simulink model "sim_all"  (R2020a)
settings: Solver=VariableStepAuto  StartTime=0.0  StopTime=2000  RelTol=1e-3
values from neighbouring files (symbols this model uses):
  a1 = rho * D^4 * alpha1    (= 0.000388302366464)    [data_current.m]
  a2 = -rho * D^3 * alpha2 * (1 - omega)    (= 0.0037030698432)    [data_current.m]
  alpha1 = 0.0113    [data_current.m]
  alpha2 = -0.0091    [data_current.m]
  cornerA = [43.781381 ... (first row only)    [missionC.m]
  cornerB = [43.780975 ... (first row only)    [missionC.m]
  cornerC = [43.780189 ... (first row only)    [missionC.m]
  cornerD = [43.780602 ... (first row only)    [missionC.m]
  ctrl_clockwise = false    [controller.m]
  ctrl_int_bound_or = 0.1    [controller.m]
  ctrl_int_bound_pos = 1    [controller.m]
  ctrl_k_or = 1    [controller.m]
  ctrl_k_pos = 1/3    (= 0.333333333333)    [controller.m]
  ctrl_Ki_vel = 100    [controller.m]
  ctrl_Kp_v_pos = 200    [controller.m]
  ctrl_Kp_vel = 200    [controller.m]
  ctrl_TAM = [  1     1           0           0               0       0;               0     0           1           1               0       0;               0     0           0           0               1       1;               0     0  -(ctrl_r+ctrl_dc)  ctrl_r+ctrl_dc    0       0;               0     0           0           0            -ctrl_r    ctrl_r;           -ctrl_r ctrl_r        0           0       ...(+19 chars)    [controller.m]
  ctrl_Ts = 0.1    [controller.m]
  ctrl_va_uncontrolled = 0.15    [controller.m]
  ctrl_vel_uncontrolled = 0.5    [controller.m]
  D = 0.076    [data_current.m]
  dead_zone_limit = 31.5    [data_current.m]
  depth = 5    [missionC.m]
  distanceFromWall = 8    [missionC.m]
  initInspectedSide = 2    [missionC.m]
  initPoint = [ 43.780796 ... (first row only)    [missionC.m]
  mod_A = pi*mod_R*mod_R    [model.m]
  mod_Cd_F = 0.45    [model.m]
  mod_Cd_M = 0.4    [model.m]
  mod_eta_init = [mod_xNorth; mod_yEast; -mod_zDown; 0; 0; 0]    [model.m]
  mod_g = 9.81    [model.m]
  mod_h0 = 0    [model.m]
  mod_Ixx = mod_Io(1,1)    [model.m]
  mod_Iyy = mod_Io(2,2)    [model.m]
  mod_Izz = mod_Io(3,3)    [model.m]
  mod_Kp_dot = 0    [model.m]
  mod_lat0 = 43.780189    [model.m]
  mod_lon0 = 11.282698    [model.m]
  mod_m = 100    [model.m]
  mod_Mq_dot = mod_Kp_dot    (= 0)    [model.m]
  mod_ni_init = [0; 0; 0; 0; 0; 0]    [model.m]
  mod_Nr_dot = mod_Kp_dot    (= 0)    [model.m]
  mod_p1 = [0; mod_R; 0]    [model.m]
  mod_p2 = [0; -mod_R; 0]    [model.m]
  mod_p3 = [0; 0; (mod_R + mod_z_cm)]    [model.m]
  mod_p4 = [0; 0; -(mod_R + mod_z_cm)]    [model.m]
  mod_p5 = [mod_R; 0; 0]    [model.m]
  mod_p6 = [-mod_R; 0; 0]    [model.m]
  mod_R = ((3*mod_Vol)/(4*pi))^(1/3)    [model.m]
  mod_Rm = (4*mod_R)/(3*pi)    [model.m]
  mod_t1 = [1; 0; 0]    [model.m]
  mod_t2 = [1; 0; 0]    [model.m]
  mod_t3 = [0; 1; 0]    [model.m]
  mod_t4 = [0; 1; 0]    [model.m]
  mod_t5 = [0; 0; 1]    [model.m]
  mod_t6 = [0; 0; 1]    [model.m]
  mod_W = mod_m*mod_g    (= 981)    [model.m]
  mod_Xu_dot = (2/3)*mod_rho_AUV*pi*(mod_R^3)    [model.m]
  mod_Yv_dot = mod_Xu_dot    [model.m]
  mod_z_cm = mod_r_cm(3)    [model.m]
  mod_Zw_dot = mod_Xu_dot    [model.m]
  n_max = 340    [data_current.m]
  nav_DT = 0.1    [navigation.m]
  nav_filter = -1    [data_analysis_simulation_total.m]    (also in navigation.m)
  nav_giro = 2    [navigation.m]
  nav_h0 = 0    [navigation.m]
  nav_lat0 = cornerC(1)    [navigation.m]
  nav_lon0 = cornerC(2)    [navigation.m]
  nav_plane_AB = coefficient_plane(nav_A,nav_B)    [navigation.m]
  nav_plane_BC = coefficient_plane(nav_B,nav_C)    [navigation.m]
  nav_plane_CD = coefficient_plane(nav_C,nav_D)    [navigation.m]
  nav_plane_DA = coefficient_plane(nav_D,nav_A)    [navigation.m]
  nav_resampling = 10000    [navigation.m]
  omega = 0.1    [data_current.m]
  relativeDirection = 30    [missionC.m]
  res_enable_n_eff = 1    [navigation.m]
  rho = 1030    [data_current.m]
  sens_distCM = 0.267    [sensors.m]
  sens_Sample_time_AHRS = 0.1    [sensors.m]
  sens_Sample_time_depth = 0.1    [sensors.m]
  sens_Sample_time_dvl = 0.2    [sensors.m]
  sens_Sample_time_GPS = 1    [sensors.m]
  sens_Sample_time_GYRO = 0.1    [sensors.m]
  sens_Sample_time_sonar = 0.5    [sensors.m]
  sens_threshold = 0.485    [sensors.m]
  sens_Variance_AHRS_pitch = (0.0087)^2    (= 7.569e-05)    [sensors.m]
  sens_Variance_AHRS_roll = (0.0087)^2    (= 7.569e-05)    [sensors.m]
  sens_Variance_AHRS_yaw = (0.0017)^2    (= 2.89e-06)    [sensors.m]
  sens_Variance_depth1 = (0.2)^2    (= 0.04)    [sensors.m]
  sens_Variance_depth2 = (0.4)^2    (= 0.16)    [sensors.m]
  sens_Variance_DVL = (speed*0.03)^2    [sensors.m]
  sens_Variance_GPS = 3    [sensors.m]
  sens_Variance_GYRO = 2.5133e-06    [sensors.m]
  sens_Variance_sonar = 0.05    [sensors.m]
  soglia_or = [0.1, 0.1, 0.1]    [mission.m]
  soglia_orp = 0.1    [mission.m]
  soglia_parete = 0.5    [mission.m]
  soglia_parete_frenata = 0.5    [mission.m]
  soglia_pos = [0.00001, 0.00001, 0.5]    [mission.m]
  soglia_SOS_collisione = 2    [mission.m]
  soglia_SOS_or = [0.25, 0.25, 0.25]    [mission.m]
  soglia_SOS_orp = 0.25    [mission.m]
  soglia_SOS_parete = 1    [mission.m]
  soglia_SOS_pos = [0.00005, 0.00005, 1]    [mission.m]
  soglia_SOS_pos_ris = 2    [mission.m]
  soglia_SOS_vel = 0.2    [mission.m]
  SOS = 0    [mission.m]
  speed = 0.4    [missionC.m]
  stato = 100    [mission.m]
  timer = 40*2    (= 80)    [mission.m]
  Ts_supervisor = 0.1    [mission.m]
undefined symbols (not defined in the file or in its folder): DiscIntNeverNeededParam, nav_A, nav_B, nav_C, nav_D
libraries: simulink x8, cstblocks x6, simulink_extras x1
(part 4 of 8)

== system sim_all/Model/Vehicle Model/P3 ==
  note: n is the rotational speed of the thruster
      | V is the speed component of the water along the thruster axis
      |
      | n is saturated according to data
      | a dead zone is considered according to data
      | the thruster is characterised by 1st order dynamics (tau = 0.2s)
  n3 [rad/s] : Inport
  V3 [m/s] : Inport  Port=2
  Dead Zone : DeadZone  LowerValue=-dead_zone_limit  UpperValue=dead_zone_limit  SaturateOnIntegerOverflow=on
  Propeller3 : MATLAB Function  TreatAsAtomicUnit=on
  Saturation : Saturate  UpperLimit=n_max  LowerLimit=-n_max
  Transfer Fcn : TransferFcn  Denominator=[0.2 1]
  T3 : Outport
  wires:
  V3 [m/s]/1 -> Propeller3/2(V3)
  Saturation/1 -> Propeller3/1(n3)
  Transfer Fcn/1 -> Saturation/1
  Dead Zone/1 -> Transfer Fcn/1
  n3 [rad/s]/1 -> Dead Zone/1
  Propeller3/1(T3) -> T3/1

== system sim_all/Model/Vehicle Model/P4 ==
  note: n is the rotational speed of the thruster
      | V is the speed component of the water along the thruster axis
      |
      | n is saturated according to data
      | a dead zone is considered according to data
      | the thruster is characterised by 1st order dynamics (tau = 0.2s)
  n4 [rad/s] : Inport
  V4 [m/s] : Inport  Port=2
  Dead Zone : DeadZone  LowerValue=-dead_zone_limit  UpperValue=dead_zone_limit  SaturateOnIntegerOverflow=on
  Propeller4 : MATLAB Function  TreatAsAtomicUnit=on
  Saturation : Saturate  UpperLimit=n_max  LowerLimit=-n_max
  Transfer Fcn : TransferFcn  Denominator=[0.2 1]
  T4 : Outport
  wires:
  V4 [m/s]/1 -> Propeller4/2(V4)
  Saturation/1 -> Propeller4/1(n4)
  Transfer Fcn/1 -> Saturation/1
  Dead Zone/1 -> Transfer Fcn/1
  n4 [rad/s]/1 -> Dead Zone/1
  Propeller4/1(T4) -> T4/1

== system sim_all/Model/Vehicle Model/P5 ==
  note: n is the rotational speed of the thruster
      | V is the speed component of the water along the thruster axis
      |
      | n is saturated according to data
      | a dead zone is considered according to data
      | the thruster is characterised by 1st order dynamics (tau = 0.2s)
  n5 [rad/s] : Inport
  V5 [m/s] : Inport  Port=2
  Dead Zone : DeadZone  LowerValue=-dead_zone_limit  UpperValue=dead_zone_limit  SaturateOnIntegerOverflow=on
  Propeller5 : MATLAB Function  TreatAsAtomicUnit=on
  Saturation : Saturate  UpperLimit=n_max  LowerLimit=-n_max
  Transfer Fcn : TransferFcn  Denominator=[0.2 1]
  T5 : Outport
  wires:
  V5 [m/s]/1 -> Propeller5/2(V5)
  Saturation/1 -> Propeller5/1(n5)
  Transfer Fcn/1 -> Saturation/1
  Dead Zone/1 -> Transfer Fcn/1
  n5 [rad/s]/1 -> Dead Zone/1
  Propeller5/1(T5) -> T5/1

== system sim_all/Model/Vehicle Model/P6 ==
  note: n is the rotational speed of the thruster
      | V is the speed component of the water along the thruster axis
      |
      | n is saturated according to data
      | a dead zone is considered according to data
      | the thruster is characterised by 1st order dynamics (tau = 0.2s)
  n6 [rad/s] : Inport
  V6 [m/s] : Inport  Port=2
  Dead Zone : DeadZone  LowerValue=-dead_zone_limit  UpperValue=dead_zone_limit  SaturateOnIntegerOverflow=on
  Propeller6 : MATLAB Function  TreatAsAtomicUnit=on
  Saturation : Saturate  UpperLimit=n_max  LowerLimit=-n_max
  Transfer Fcn : TransferFcn  Denominator=[0.2 1]
  T6 : Outport
  wires:
  V6 [m/s]/1 -> Propeller6/2(V6)
  Saturation/1 -> Propeller6/1(n6)
  Transfer Fcn/1 -> Saturation/1
  Dead Zone/1 -> Transfer Fcn/1
  n6 [rad/s]/1 -> Dead Zone/1
  Propeller6/1(T6) -> T6/1

== system sim_all/PF/Particle Filter/AHRS__check ==
  AHRS_new : Inport
  MATLAB Function4 : MATLAB Function  TreatAsAtomicUnit=on
  Memory4 : Memory
  flag_AHRS : Outport
  AHRS_now : Outport  Port=2
  wires:
  AHRS_new/1 -> MATLAB Function4/1(AHRS_new)
  Memory4/1 -> MATLAB Function4/2(AHRS_old)
  MATLAB Function4/1(flag_AHRS) -> flag_AHRS/1
  MATLAB Function4/2(AHRS_now) -> Memory4/1, AHRS_now/1

== system sim_all/PF/Particle Filter/CORREZIONE ==
  x : Inport
  P : Inport  Port=2
  s : Inport  Port=3
  w_k : Inport  Port=4
  flag : Inport  Port=5
  nav_flag_init : Inport  Port=6
  MATLAB Function : MATLAB Function  TreatAsAtomicUnit=on  SystemSampleTime=nav_DT
  x_k+1 : Outport  PortDimensions=[3 1]
  P_ : Outport  Port=2  PortDimensions=[3 3]
  "s " : Outport  Port=3
  w : Outport  Port=4
  wires:
  x/1 -> MATLAB Function/1(x_k_1)
  P/1 -> MATLAB Function/2(P_k_1)
  s/1 -> MATLAB Function/3("s ")
  w_k/1 -> MATLAB Function/4("w ")
  flag/1 -> MATLAB Function/5(flag)
  MATLAB Function/1(x) -> x_k+1/1
  MATLAB Function/2(P) -> P_/1
  MATLAB Function/3(s) -> "s "/1
  MATLAB Function/4(w) -> w/1
  nav_flag_init/1 -> MATLAB Function/6(nav_flag_init)

== system sim_all/PF/Particle Filter/DVL_check ==
  DVL_new : Inport
  MATLAB Function4 : MATLAB Function  TreatAsAtomicUnit=on
  Memory4 : Memory
  flag_DVL : Outport
  DVL_now : Outport  Port=2
  wires:
  DVL_new/1 -> MATLAB Function4/1(DVL_new)
  Memory4/1 -> MATLAB Function4/2(DVL_old)
  MATLAB Function4/1(flag_DVL) -> flag_DVL/1
  MATLAB Function4/2(DVL_now) -> Memory4/1, DVL_now/1

== system sim_all/PF/Particle Filter/MISURA VIRTUALE ==
  s : Inport
  w : Inport  Port=2
  flag_vect : Inport  Port=3
  mis_vect : Inport  Port=4
  J : Inport  Port=5
  R : Inport  Port=6
  MATLAB Function : MATLAB Function  TreatAsAtomicUnit=on  SystemSampleTime=nav_DT
  w_k : Outport
  flag : Outport  Port=2
  wires:
  MATLAB Function/1(w_k) -> w_k/1
  MATLAB Function/2(flag) -> flag/1
  s/1 -> MATLAB Function/1(s)
  w/1 -> MATLAB Function/2(w)
  flag_vect/1 -> MATLAB Function/3(flag_vect)
  mis_vect/1 -> MATLAB Function/4(mis_vect)
  J/1 -> MATLAB Function/5(J)
  R/1 -> MATLAB Function/6(R)

== system sim_all/PF/Particle Filter/PREDIZIONE ==
  s0 : Inport
  w0 : Inport  Port=2
  "s " : Inport  Port=3
  w : Inport  Port=4
  DVL : Inport  Port=5
  orient : Inport  Port=6
  Q : Inport  Port=7
  "nav_flag_init " : Inport  Port=8
  MATLAB Function : MATLAB Function  TreatAsAtomicUnit=on  SystemSampleTime=nav_DT
  x : Outport
  P : Outport  Port=2
  s : Outport  Port=3
  W : Outport  Port=4
  nav_flag_init : Outport  Port=5
  wires:
  MATLAB Function/4(w) -> W/1
  MATLAB Function/2(P) -> P/1
  w0/1 -> MATLAB Function/2(w0)
  MATLAB Function/1(x) -> x/1
  s0/1 -> MATLAB Function/1(s0)
  orient/1 -> MATLAB Function/5(orient)
  DVL/1 -> MATLAB Function/6(DVL)
  "s "/1 -> MATLAB Function/3("s ")
  MATLAB Function/3(s) -> s/1
  MATLAB Function/5(nav_flag_init) -> nav_flag_init/1
  Q/1 -> MATLAB Function/7(Q)
  "nav_flag_init "/1 -> MATLAB Function/8("nav_flag_init ")
  w/1 -> MATLAB Function/4("w ")

== system sim_all/PF/Particle Filter/Q_error ==
  flag_AHRS : Inport
  flag_DVL : Inport  Port=2
  Q : Inport  Port=3
  MATLAB Function4 : MATLAB Function  TreatAsAtomicUnit=on
  Memory : Memory
  Q_k : Outport
  wires:
  MATLAB Function4/1(Q_k) -> Q_k/1, Memory/1
  flag_AHRS/1 -> MATLAB Function4/3(flag_AHRS)
  flag_DVL/1 -> MATLAB Function4/4(flag_DVL)
  Memory/1 -> MATLAB Function4/2(Q_k_1)
  Q/1 -> MATLAB Function4/1(Q)

== system sim_all/PF/Particle Filter/RICAMPIONAMENTO ==
  "s " : Inport
  w : Inport  Port=2
  Constant : Constant  Value=res_enable_n_eff
  MATLAB Function : MATLAB Function  TreatAsAtomicUnit=on
  Pulse Generator : DiscretePulseGenerator  PulseType=Time based  Period=nav_resampling  PhaseDelay=nav_resampling
  Scope : Scope  Commented=on
  Scope1 : Scope  Commented=on
  s_new : Outport
  w_new : Outport  Port=2
  wires:
  MATLAB Function/2(w_new) -> w_new/1
  MATLAB Function/1(s_new) -> s_new/1
  "s "/1 -> MATLAB Function/1(s)
  w/1 -> MATLAB Function/2(w)
  Pulse Generator/1 -> MATLAB Function/3(pulse)  "resampling pulse"
  MATLAB Function/3(n_eff) -> Scope/1  "n_eff"
  MATLAB Function/4(n_eff_pulse) -> Scope1/1  "n_eff_pulse"
  Constant/1 -> MATLAB Function/4(en)

== system sim_all/Sensors/BLOCCO GYRO1/Subsystem ==
  t : Inport  SampleTime=sens_Sample_time_GYRO
  GEOD to NED : MATLAB Function  TreatAsAtomicUnit=on
  Bias_G : Outport
  wires:
  t/1 -> GEOD to NED/1(t)
  GEOD to NED/1(Bias_G) -> Bias_G/1

== matlab function sim_all/Mission_supervisor_v3/Mission_Supervisor/Risalita/MATLAB Function ==
  data: delta_SOS input; delta_current_ris output; delta_stato_ris output; Pos_d output size=3; Dpp_d output; Dps_d output; Pos_s input; Dpp_s input; Orp_s input; Dps_s input; distanceFromWall parameter; Orp_d output; relativeDirection parameter; soglia_pos parameter; SOS parameter; Dps_fin input; soglia_SOS_pos_ris parameter; soglia_SOS_orp parameter; error_flag input; SOS_205 input; initPoint parameter; soglia_SOS_collisione parameter
function [delta_current_ris, delta_stato_ris, Pos_d, Dpp_d, Dps_d, Orp_d ] = Risalita(delta_SOS, Pos_s, Dpp_s, Orp_s, Dps_s, distanceFromWall, relativeDirection, soglia_pos, SOS, Dps_fin, soglia_SOS_pos_ris, soglia_SOS_orp, error_flag, SOS_205, initPoint, soglia_SOS_collisione)

    disp("Risalita");
    
    %% Unità di misura 
    
    % Pos_d, Pos_s, soglia_pos, initPoint                                                                      [deg,deg,m]
    % Orp_d, Orp_s, soglia_SOS_orp                                                                             [rad]
    % relativeDirection                                                                                        [deg]
    % Dpp_d, Dps_d, Dpp_s, Dps_s, Dps_fin, distanceFromWall, soglia_SOS_collisione_s, soglia_SOS_collisione    [m]

    %% Inizializzazione variabili
    
    delta_stato_ris = 0;
    
    pronti = false; 
    
    %% Preparazione dei riferimenti da fornire ai blocchi successivi
    
    % Posizione da raggiungere
    Pos_d = [nan; nan; initPoint(3)];
    
    % Distanza da mantenere
    Dpp_d = distanceFromWall;
    Dps_d = Dps_fin;
    
    % Orientazione da mantenere
    Orp_d = deg2rad(relativeDirection);
    
    % Transizione di stato effettiva
    delta_current_ris = 301 - delta_SOS;  
    
    
    %% Verifica
    
    % Verifica sull'orientazione rispetto alla parete
    if (abs(Orp_s - Orp_d) > soglia_SOS_orp)
        
        SOS = 1;
        disp("EMERGENZA: Rilevato errore nell'orientazione relativa da parete");
        
    end
                                                                            %******TEST******
                                                                            %test = 30;
    % In base al meccanismo del "gestore dell'emergenza" si distinguono due casi: 
    % uno in cui lo stato di Risalita viene attivato al termine di un 
    % pattugliamento corretto (la codifica dello stato precedente è pari a 205) 
    % ed uno se la transizione in questo stato è dovuta all'aver
    % intrapreso una manovra di emergenza (lo stato precedente è
    % inferiore a 205).
    
    % Si proviene da un pattugliamento senza emergenza e si verifica di 
    % effettuare la risalita nella posizione giusta
    if (delta_SOS == 205 && SOS_205 == 0)
        if (abs(Dpp_s - Dpp_d) > soglia_SOS_pos_ris || ...                                          
            abs(Dps_s - Dps_fin) > soglia_SOS_pos_ris)
             
            SOS = 1;
            disp("EMERGENZA: Avvicinamento eccessivo alla parete");
            
        end
    
    % Si proviene da una situazione di emergenza oppure l'emergenza avviene in
    % "risalita". Verifica di effettuare la risalita senza collisione
    % con le pareti
    elseif (delta_SOS < 205 || SOS_205 == 1)
        
        if (abs(Dpp_s - Dpp_d) > soglia_SOS_collisione || ...
            abs(Dps_s) < soglia_SOS_collisione)
       
            SOS = 1;
            disp("EMERGENZA: Avvicinamento eccessivo alla parete");
            
        end
        
    end
    
    if error_flag == 1
        disp("EMERGENZA: Errore segnalato dagli altri sottosistemi");
        SOS = 1;
    end
    
                                                                            %*****TEST******% 
                                                                            %Dps_fin = 8;

    % Si verifica di aver raggiunto la superficie
    if (SOS == 0 && ... 
        abs(Pos_s(3) - Pos_d(3)) < soglia_pos(3)) 
    
          pronti = true;
        
    end
    
    
    %% Decisione dello stato successivo
    
    if ((pronti == true && (delta_SOS < 205 || SOS_205 == 1) || ...
        (SOS == 1)))
           
           delta_stato_ris = 304 - 301; % Transizione nello stato finale a causa di emergenza
    else
        if pronti == true
            
            delta_stato_ris = 302 - 301; % Transizione eseguita correttamente
        end
    end
    % Si rimane nello stato corrente
     
end

== matlab function sim_all/Controller_mk4_v3/lld2Ned1 ==
  data: x_ecef input size=[3 1]; x_n output; cornerC parameter
%% Da LLD (stima posizione assoluta) a NED
function x_n = ToNed_Pos(x_ecef,cornerC)
x_n=zeros(3,1);
coder.extrinsic('evalin', 'wgs84Ellipsoid', 'geodetic2ned');
[pNorth,pEast,pDown] = geodetic2ned(x_ecef(1),x_ecef(2),x_ecef(3),cornerC(1),cornerC(2),0,wgs84Ellipsoid);
x_n=[pNorth;pEast;x_ecef(3)];

end

== matlab function sim_all/Sensors/Environment and Sensors Model3/MATLAB Function1 ==
  data: pos input; plane_AB input; plane_BC input; plane_CD input; plane_DA input; plane_W input; dist output; Roll input; Pitch input; Yaw input
function dist = inter(pos,plane_AB,plane_BC,plane_CD,plane_DA,plane_W,Roll,Pitch, Yaw)
Nc=3; %numero di campioni per 'croce' di raggio del cono
WBr=deg2rad(5); % ampiezza semifascio del sonar (fascio considerato di 10°)
dist2=zeros(3,3);
R=linspace(Roll-WBr,Roll+WBr,Nc);
P=Pitch;
Y=linspace(Yaw-WBr, Yaw+WBr,Nc);
for j=1:Nc  %costruisco la croce (doppia)
for i=1:Nc
    
R_x = [1        0              0; %roll
      0 cos(R(i))  sin(R(i));
      0 -sin(R(i)) cos(R(i))];
  
R_y = [cos(P) 0 -sin(P); %pitch
          0           1         0;
       sin(P) 0 cos(P)];
   
R_z = [cos(Y(j)) sin(Y(j)) 0; %yaw
      -sin(Y(j)) cos(Y(j)) 0;
          0                 0        1];
      
jaco = (R_z'*R_y');
jacob = jaco*R_x';

    versore_son_body = [0 1 0]';
    versore_son_NED = jacob*versore_son_body;         %versore terna NED sonar prua

    %imposto il sistema per trovare l'intersezione tra la retta con direzione
    %nota e uno dei piani delle pareti del bacino

    t_AB = -(pos(1)+plane_AB(2)*pos(2)+plane_AB(4))/(plane_AB(2)*versore_son_NED(2)+versore_son_NED(1));
    t_BC = -(pos(1)+plane_BC(2)*pos(2)+plane_BC(4))/(plane_BC(2)*versore_son_NED(2)+versore_son_NED(1));
    t_CD = -(pos(1)+plane_CD(2)*pos(2)+plane_CD(4))/(plane_CD(2)*versore_son_NED(2)+versore_son_NED(1));
    t_DA = -(pos(1)+plane_DA(2)*pos(2)+plane_DA(4))/(plane_DA(2)*versore_son_NED(2)+versore_son_NED(1));
    t_W = -(plane_W(3)*pos(3)/(plane_W(3)*versore_son_NED(3)+versore_son_NED(3)));
    
    
    if t_AB < 0
        t_AB = inf;
    end
    if t_BC < 0
        t_BC = inf;
    end
    if t_CD < 0
        t_CD = inf;
    end
    if t_DA < 0
        t_DA = inf;
    end
    if t_W < 0
        t_W = inf;
    end
           dist1 = min([t_AB t_BC t_CD t_DA t_W]);
           
           if dist1==t_W %se incontro l'acqua metto NaN nella misura delle distanze
               dist2(i,j)=NaN;
           else
               dist2(i,j)=dist1;
           end
           
end
end
    contr=isnan(dist2); %controlla la presenza di NaN nel vettore di misure
    sum1=sum(sum(contr)); % conta il numero di NaN presenti
    
    if sum1>4 %incontro un numero di Nan superiore a 4
        dist=NaN;
    else
        dist=mean(nanmean(dist2));
    end
end

== matlab function sim_all/Mission_supervisor_v3/Mission_Supervisor/Orientazione Iniziale/MATLAB Function ==
  data: delta_stato_or_iniz output; delta_current_or_iniz output; Pos_d output size=3; Pos_s input size=3; Or_s input size=3; Or_in input; initPoint parameter size=3; Or_d output size=3; error_flag input; soglia_or parameter; soglia_SOS_pos parameter; SOS parameter; soglia_SOS_or parameter
function [delta_stato_or_iniz, delta_current_or_iniz, Pos_d, Or_d] = Orientazione_iniziale(Pos_s, Or_s, Or_in, initPoint, error_flag, soglia_or, soglia_SOS_pos, SOS, soglia_SOS_or)

    disp("Orientazione iniziale");
    
    %% Unità di misura 
    
    % Pos_d, Pos_s, initPoint, soglia_SOS_pos                                [deg, deg, m]
    % Or_d, Or_s, Or_in, soglia_or, soglia_SOS_or                            [rad, rad, rad]
    
    %% Inizializzazione variabili
    
    % Mantenimento dello stato_interno al valore
    % desiderato durante la permanenza del sistema nello stato corrente.
    delta_stato_or_iniz = 0;
    
    % Variabile utilizzata per segnalare il momento in cui
    % effettuare la transizione di stato. 
    pronti = false;
    
    %% Preparazione dei riferimenti da fornire ai blocchi successivi
                
    % Posizione da mantenere
    Pos_d = initPoint; 
   
    % Orientazione desiderata per raggiungere
    % il punto di inizio pattugliamento
    Or_d = Or_in;
    
    % Quando i riferimenti sono correttamente settati
    % il passaggio di stato viene comunicato agli altri moduli
    delta_current_or_iniz = 101 - 100;
    
    
    %% Verifiche
    
    % Si verifica il mantenimento della posizione 
    % e la ricezione della stima di orientazione
    if (abs(Pos_s(1) - Pos_d(1)) > soglia_SOS_pos(1) || ...
        abs(Pos_s(2) - Pos_d(2)) > soglia_SOS_pos(2) || ...
        abs(Pos_s(3) - Pos_d(3)) > soglia_SOS_pos(3) || ...
        isnan(Or_s(1)) || isnan(Or_s(2)) || isnan(Or_s(3)) || ...
        abs(Or_s(1) - Or_d(1)) > soglia_SOS_or(1) || ...
        abs(Or_s(2) - Or_d(2)) > soglia_SOS_or(2))
    
        SOS = 1;
        disp("EMERGENZA:");
        
        if (abs(Pos_s(1) - Pos_d(1)) > soglia_SOS_pos(1))
            disp("Rilevato errore sulla posizione X");
        end
        if (abs(Pos_s(2) - Pos_d(2)) > soglia_SOS_pos(2))
            disp("Rilevato errore sulla posizione Y");
        end
        if (abs(Pos_s(3) - Pos_d(3)) > soglia_SOS_pos(3))
            disp("Rilevato errore sulla profondita Z");
        end
        if (isnan(Or_s(1)))
            disp("Mancata ricezione della prima componente di orientazione");
        end
        if (isnan(Or_s(2)))
            disp("Mancata ricezione della seconda componente di orientazione");
        end
        if (isnan(Or_s(3)))
            disp("Mancata ricezione della terza componente di orientazione");
        end
        if (abs(Or_s(1) - Or_d(1)) > soglia_SOS_or(1))
            disp("Rilevato errore sulla rotazione di roll");
        end
        if (abs(Or_s(2) - Or_d(2)) > soglia_SOS_or(2))
            disp("Rilevato errore sulla rotazione di pitch");
        end
    end

    if error_flag == 1
        disp("EMERGENZA: errore segnalato dagli altri sottosistemi");
        SOS = 1;
    end
    
    % Si verifica di aver raggiunto l'orientazione desiderata
    if (SOS == 0 && ...
        (abs(Or_s(3) - Or_d(3)) < soglia_or(3)))
    
        pronti = true;
        
    end
       
    %% Decisione dello stato successivo
    
    if pronti == true
        
        delta_stato_or_iniz = 102 - 101; % Transizione eseguita correttamente
    end
        
    if SOS == 1
            
            delta_stato_or_iniz = 304 - 101; % Transizione nello stato di emergenza
    end
    % Si rimane nello stato corrente

end

== matlab function sim_all/Sensors/Environment and Sensors Model4/MATLAB Function1 ==
  data: pos input size=[3]; plane_AB input; plane_BC input; plane_CD input; plane_DA input; plane_W input; dist output; Roll input; Pitch input; Yaw input
function dist = inter(pos,plane_AB,plane_BC,plane_CD,plane_DA,plane_W,Roll,Pitch, Yaw)
Nc=3; %numero di campioni per 'croce' di raggio del cono=1
WBr=deg2rad(5); % ampiezza semifascio del sonar (fascio considerato di 10°)
dist2=zeros(3,3);
R=linspace(Roll-WBr,Roll+WBr,Nc);
P=Pitch;
Y=linspace(Yaw-WBr, Yaw+WBr,Nc);
for j=1:Nc  %costruisco la croce (doppia)
for i=1:Nc
    
R_x = [1        0              0; %roll
      0 cos(R(i))  sin(R(i));
      0 -sin(R(i)) cos(R(i))];
  
R_y = [cos(P) 0 -sin(P); %pitch
          0           1         0;
       sin(P) 0 cos(P)];
   
R_z = [cos(Y(j)) sin(Y(j)) 0; %yaw
      -sin(Y(j)) cos(Y(j)) 0;
          0                 0        1];
      
jaco = (R_z'*R_y');
jacob = jaco*R_x';

    versore_son_body = [0 -1 0]';
    versore_son_NED = jacob*versore_son_body;         %versore terna NED sonar prua

    %imposto il sistema per trovare l'intersezione tra la retta con direzione
    %nota e uno dei piani delle pareti del bacino

    t_AB = -(pos(1)+plane_AB(2)*pos(2)+plane_AB(4))/(plane_AB(2)*versore_son_NED(2)+versore_son_NED(1));
    t_BC = -(pos(1)+plane_BC(2)*pos(2)+plane_BC(4))/(plane_BC(2)*versore_son_NED(2)+versore_son_NED(1));
    t_CD = -(pos(1)+plane_CD(2)*pos(2)+plane_CD(4))/(plane_CD(2)*versore_son_NED(2)+versore_son_NED(1));
    t_DA = -(pos(1)+plane_DA(2)*pos(2)+plane_DA(4))/(plane_DA(2)*versore_son_NED(2)+versore_son_NED(1));
    t_W = -(plane_W(3)*pos(3)/(plane_W(3)*versore_son_NED(3)+versore_son_NED(3)));
    
    
    if t_AB < 0
        t_AB = inf;
    end
    if t_BC < 0
        t_BC = inf;
    end
    if t_CD < 0
        t_CD = inf;
    end
    if t_DA < 0
        t_DA = inf;
    end
    if t_W < 0
        t_W = inf;
    end
           dist1 = min([t_AB t_BC t_CD t_DA t_W]);
           
           if dist1==t_W %se incontro l'acqua metto NaN nella misura delle distanze
               dist2(i,j)=NaN;
           else
               dist2(i,j)=dist1;
           end
           
end
end
    contr=isnan(dist2); %controlla la presenza di NaN nel vettore di misure
    sum1=sum(sum(contr)); % conta il numero di NaN presenti
    
    if sum1>4 %incontro un numero di Nan superiore a 4
        dist=NaN;
    else
        dist=mean(nanmean(dist2));
    end
end

== matlab function sim_all/Sensors/Environment and Sensors Model6/MATLAB Function1 ==
  data: pos input; plane_AB input; plane_BC input; plane_CD input; plane_DA input; plane_W input; dist output; Roll input; Pitch input; Yaw input
function dist = inter(pos,plane_AB,plane_BC,plane_CD,plane_DA,plane_W,Roll,Pitch, Yaw)
Nc=3; %numero di campioni per 'croce' di raggio del cono
WBr=deg2rad(5); % ampiezza semifascio del sonar (fascio considerato di 10°)
dist2=zeros(3,3);
R=Roll;
P=linspace(Pitch-WBr,Pitch+WBr,Nc);
Y=linspace(Yaw-WBr, Yaw+WBr,Nc);

for j=1:Nc  %costruisco la croce (doppia)
for i=1:Nc
    
R_x = [1        0              0; %roll
      0 cos(R)  sin(R);
      0 -sin(R) cos(R)];
  
R_y = [cos(P(i)) 0 -sin(P(i)); %pitch
          0           1         0;
       sin(P(i)) 0 cos(P(i))];
   
R_z = [cos(Y(j)) sin(Y(j)) 0; %yaw
      -sin(Y(j)) cos((j)) 0;
          0                 0        1];
      
jaco = (R_z'*R_y');
jacob = jaco*R_x';

    versore_son_body = [1 0 0]'; %prua
    versore_son_NED = jacob*versore_son_body;         %versore terna NED sonar prua

    %imposto il sistema per trovare l'intersezione tra la retta con direzione
    %nota e uno dei piani delle pareti del bacino

    t_AB = -(pos(1)+plane_AB(2)*pos(2)+plane_AB(4))/(plane_AB(2)*versore_son_NED(2)+versore_son_NED(1));
    t_BC = -(pos(1)+plane_BC(2)*pos(2)+plane_BC(4))/(plane_BC(2)*versore_son_NED(2)+versore_son_NED(1));
    t_CD = -(pos(1)+plane_CD(2)*pos(2)+plane_CD(4))/(plane_CD(2)*versore_son_NED(2)+versore_son_NED(1));
    t_DA = -(pos(1)+plane_DA(2)*pos(2)+plane_DA(4))/(plane_DA(2)*versore_son_NED(2)+versore_son_NED(1));
    t_W = -(plane_W(3)*pos(3)/(plane_W(3)*versore_son_NED(3)+versore_son_NED(3)));
    
    
    if t_AB < 0
        t_AB = inf;
    end
    if t_BC < 0
        t_BC = inf;
    end
    if t_CD < 0
        t_CD = inf;
    end
    if t_DA < 0
        t_DA = inf;
    end
    if t_W < 0
        t_W = inf;
    end
           dist1 = min([t_AB t_BC t_CD t_DA t_W]);
           
           if dist1==t_W %se incontro l'acqua metto NaN nella misura delle distanze
               dist2(i,j)=NaN;
           else
               dist2(i,j)=dist1;
           end
           
end
end
    contr=isnan(dist2); %controlla la presenza di NaN nel vettore di misure
    sum1=sum(sum(contr)); % conta il numero di NaN presenti
    
    if sum1>4 %incontro un numero di Nan superiore a 4
        dist=NaN;
    else
        dist=mean(nanmean(dist2));
    end
end

== matlab function sim_all/Sensors/Environment1 ==
  data: plane_AB output; plane_BC output; plane_CD output; plane_DA output; plane_W output
function [plane_AB,plane_BC,plane_CD,plane_DA,plane_W] = fcn()
%% Inizializzazione
% Coordinate degli spigoli del bacino in lat e long fornite dal file
% missionC.m
A= zeros(1,3);
B= zeros(1,3);
C= zeros(1,3);
D= zeros(1,3);
cornerA = [43.781381; 11.282793]; % Lat/Lon [decimal degrees]      
cornerB = [43.780975; 11.283505]; % Lat/Lon [decimal degrees]       
cornerC = [43.780189; 11.282698]; % Lat/Lon [decimal degrees]       
cornerD = [43.780602; 11.281956]; % Lat/Lon [decimal degrees]

% Definizione terna NED con origine (lat0,long0,h0) coincidente al 
% cornerD
coder.extrinsic('evalin', 'wgs84Ellipsoid', 'geodetic2ned');
lat0 = cornerC(1);
lon0 = cornerC(2);
h0 = 0;

%% Conversione ECEF to NED
[A(1),A(2),A(3)] = geodetic2ned(cornerA(1),cornerA(2),0,lat0,lon0,h0,wgs84Ellipsoid);
[B(1),B(2),B(3)] = geodetic2ned(cornerB(1),cornerB(2),0,lat0,lon0,h0,wgs84Ellipsoid);
[C(1),C(2),C(3)] = geodetic2ned(cornerC(1),cornerC(2),0,lat0,lon0,h0,wgs84Ellipsoid);
[D(1),D(2),D(3)] = geodetic2ned(cornerD(1),cornerD(2),0,lat0,lon0,h0,wgs84Ellipsoid);

%% Calcolo delle distanze dalle pareti
% L'equazione del piano corrisponde a quella della retta perché il piano
% delle pareti è verticale, per cui si risolve un sistema lineare:
% l'equazione del piano deve soddisfare il passaggio da due punti.
% Il parametro a è libero, lo poniamo a=1, il parametro c relativo all'asse
% z sarà sempre pari a zero.

% questo è il sistema da risolvere
b = - (B(1)- A(1)) /( B(2) - A(2) );   %AB
d = - A(1) - A(2)*b;

e = - (C(1)-B(1))/(C(2)-B(2));         %BC
f = - B(1) - B(2)*e;

g = - (D(1) - C(1)) / (D(2) - C(2));   %CD
h = - C(1) - C(2)*g;

i = - (A(1) - D(1))/(A(2) - D(2));     %DA
l = -D(1) - D(2)*i;

% syms b d;
% [b d] = solve(A(1)+b*A(2)+d,B(1)+b*B(2)+d,b,d);
a_AB = 1;
b_AB = double(b);
c_AB = 0;
d_AB = double(d);
% 
% syms b d ;
% [b d] = solve(B(1)+b*B(2)+d,C(1)+b*C(2)+d,b,d);
a_BC = 1;
b_BC = double(e);
c_BC = 0;
d_BC = double(f);

a_CD = 1;
b_CD = double(g);
c_CD = 0;
d_CD = double(h);

a_DA = 1;
b_DA = double(i);
c_DA = 0;
d_DA = double(l);


% calcolo dei coefficienti del piano direttamente con la formula esplicita
plane_AB = [a_AB b_AB c_AB d_AB];
plane_BC = [a_BC b_BC c_BC d_BC];
plane_CD = [a_CD b_CD c_CD d_CD];
plane_DA = [a_DA b_DA c_DA d_DA];
plane_W =[0 0 1 0];

== matlab function sim_all/Sensors/GEOD to NED1 ==
  data: z output; lat input; lon input; h input
function z  = fcn(lat,lon,h)
z=[0;0;0];
coder.extrinsic('evalin','wgs84Ellipsoid','geodetic2ned');
[N,E,D] = geodetic2ned(lat,lon,h,43.780189,11.282698,0,wgs84Ellipsoid);
z=[N;E;D];

== matlab function sim_all/Sensors/NED to GEOD1 ==
  data: z output; N input; E input
function z  = fcn(N,E)
z=zeros(2,1);
coder.extrinsic('evalin','wgs84Ellipsoid','ned2geodetic');
%profondità considerata come solo antenna GPS fuori dall'acqua
[LAT,LON,~]=ned2geodetic(N,E,-0.385,43.780189,11.282698,0,wgs84Ellipsoid);
z=[LAT;LON];

== matlab function sim_all/Model/from Rad to Deg ==
  data: eta2 input; eta2_deg output
function eta2_deg = fcn(eta2)

phi = eta2(1);
theta = eta2(2);
psi = eta2(3);

% Si effettua una conversione da radianti a gradi dell'angolo di roll:
k_phi = fix(phi/(2*pi));
orientation_phi = phi - (2*pi*k_phi);
phi_deg = (180*orientation_phi)/pi;

% Si effettua una conversione da radianti a gradi dell'angolo di pitch:
k_theta = fix(theta/(2*pi));
orientation_theta = theta - (2*pi*k_theta);
theta_deg = (180*orientation_theta)/pi;

% Si effettua una conversione da radianti a gradi dell'angolo di yaw:
k_psi = fix(psi/(2*pi));
orientation_psi = psi - (2*pi*k_psi);
psi_deg = (180*orientation_psi)/pi;

% Se si vuole mostrare anche il numero di rotazioni che compie il robot in
% roll, pitch o yaw mandare in uscita anche k_phi, k_theta e k_psi.

eta2_deg = [phi_deg; theta_deg; psi_deg];

== matlab function sim_all/Controller_mk4_v3/signal_to_NED/Signal_d->NED/ToNed ==
  data: vel input; ddp input; dps input; orp input; vel_n output size=[3 1]; wall_vect input; wall_vect2 input; state input; ctrl_clockwise parameter; ddp_n output size=[3 1]; dps_n output size=[3 1]; orp_n output size=[3 1]
%% A partire dai riferimenti scalari calcola i relativi vettori in terna NED
function [vel_n,ddp_n,dps_n,orp_n] = ToNed(vel, ddp, dps, orp, wall_vect, wall_vect2, state, ctrl_clockwise)
    w=wall_vect/norm(wall_vect);        % versore relativo alla pareta che stiamo pattugliando
    n = Cz(-pi/2)*wall_vect;            % vettore ortogonale entrante dalla parete in pattugliamento
    n=n/norm(n);                        % versore ortogonale alla parete in pattugliamento
    n2 = Cz(-pi/2)*wall_vect2;          % vettore ortogonale entrante dalla parete successiva
    n2=n2/norm(n2);                     % versore ortogonale alla parete successiva
    if ctrl_clockwise == true           % la velocità dipende dalla direzione di pattugliamento
        vel_n=w*vel;                    % stessa direzione della parete
    else
        vel_n=-w*vel;
    end
    ddp_n = n*ddp;                          % vettore distanza dalla parete in pattugliamento in ned
    dps_n = n2*dps;                         % vettore distanza dalla parete successiva in ned
    v_orp = -n;                             % deve essere uscente dal bacino
    v_orp = Cz(-orp)*v_orp;                 % ruoto dell' angolo di riferimento
    orp_n=[0;0;atan2(v_orp(2),v_orp(1))];   % angolo rispetto all'asse x della terna ned
    if(state == 203)                        % orp_n deve essere relativo alla parete successiva
        v_orp = -n2;
        v_orp = Cz(-orp)*v_orp;
        orp_n=[0;0;atan2(v_orp(2),v_orp(1))];
    end
end

== matlab function sim_all/Controller_mk4_v3/signal_to_NED/Signal_d->NED/wall_fcn ==
  data: wall_vect output; WALL input; cornerA parameter; cornerB parameter; cornerC parameter; cornerD parameter; wall_vect2 output; ctrl_clockwise parameter
%% Restituisce i vettori Parete in pattugliamento e Parete successiva
function [wall_vect, wall_vect2] = wall_fcn(WALL,cornerA, cornerB, cornerC, cornerD, ctrl_clockwise) %inspectionDirection
    AB = zeros(3,1);
    BC = zeros(3,1);
    CD = zeros(3,1);
    DA = zeros(3,1);
    a = zeros(3,1);
    b = zeros(3,1);
    c = zeros(3,1);
    d = zeros(3,1);
    coder.extrinsic('evalin', 'wgs84Ellipsoid', 'geodetic2ned');
    [aNorth,aEast,aDown] = geodetic2ned(cornerA(1),cornerA(2),0,cornerC(1),cornerC(2),0,wgs84Ellipsoid);
    [bNorth,bEast,bDown] = geodetic2ned(cornerB(1),cornerB(2),0,cornerC(1),cornerC(2),0,wgs84Ellipsoid);
    [cNorth,cEast,cDown] = geodetic2ned(cornerC(1),cornerC(2),0,cornerC(1),cornerC(2),0,wgs84Ellipsoid);
    [dNorth,dEast,dDown] = geodetic2ned(cornerD(1),cornerD(2),0,cornerC(1),cornerC(2),0,wgs84Ellipsoid);
    a=[aNorth;aEast;aDown];
    b=[bNorth;bEast;bDown];
    c=[cNorth;cEast;cDown];
    d=[dNorth;dEast;dDown];
    AB = b-a;
    BC = c-b;
    CD = d-c;
    DA = a-d;
    if WALL == 1
        wall_vect = AB;
        if ctrl_clockwise == true
            wall_vect2 = BC;
        else
            wall_vect2 = DA;
        end
    elseif WALL == 2
        wall_vect = BC;
        if ctrl_clockwise == true
            wall_vect2 = CD;
        else
            wall_vect2 = AB;
        end
    elseif  WALL == 3
        wall_vect = CD;
        if ctrl_clockwise == true
            wall_vect2 = DA;
        else
            wall_vect2 = BC;
        end
    else   
        wall_vect = DA;
        if ctrl_clockwise == true
            wall_vect2 = AB;
        else
            wall_vect2 = CD;
        end
    end
end

== matlab function sim_all/Controller_mk4_v3/C_or/eta_dot2ni ==
  data: eta_dot input; or input; va output
%% Da NED a BODY
function va = fcn(eta_dot, or)

phi= or(1);
theta= or(2); 
psi= or(3);

J2inv = [[1;0;0], Cx(phi)*[0;1;0], Cx(phi)*Cy(theta)*[0;0;1]];
va = J2inv * eta_dot;
end

== matlab function sim_all/Controller_mk4_v3/signal_to_NED/Signal_s->NED/ToNed ==
  data: ddp input; dps input; wall_vect input; ddp_n output size=[3 1]; dps_n output size=[3 1]; wall_vect2 input
%% A partire dalle stime scalari calcola i relativi vettori in terna NED
function [ddp_n,dps_n] = ToNed_s(ddp, dps,wall_vect, wall_vect2)
    n = Cz(-pi/2)*wall_vect;            % vettore ortogonale entrante dalla parete in pattugliamento
    n=n/norm(n);                        % versore ortogonale alla parete in pattugliamento
    n2 = Cz(-pi/2)*wall_vect2;          % vettore ortogonale entrante dalla parete successiva
    n2=n2/norm(n2);                     % versore ortogonale alla parete successiva
    ddp_n = n*ddp;                      % vettore distanza dalla parete in pattugliamento in ned
    dps_n = n2*dps;                     % vettore distanza dalla parete successiva in ned
end

== matlab function sim_all/Controller_mk4_v3/signal_to_NED/Signal_s->NED/wall_fcn1 ==
  data: wall_vect output; WALL input; cornerA parameter; cornerB parameter; cornerC parameter; cornerD parameter; wall_vect2 output; ctrl_clockwise parameter
%% Restituisce i vettori Parete in pattugliamento e Parete successiva
function [wall_vect, wall_vect2] = wall_fcn(WALL,cornerA, cornerB, cornerC, cornerD, ctrl_clockwise) %inspectionDirection
    AB = zeros(3,1);
    BC = zeros(3,1);
    CD = zeros(3,1);
    DA = zeros(3,1);
    a = zeros(3,1);
    b = zeros(3,1);
    c = zeros(3,1);
    d = zeros(3,1);
    coder.extrinsic('evalin', 'wgs84Ellipsoid', 'geodetic2ned');
    [aNorth,aEast,aDown] = geodetic2ned(cornerA(1),cornerA(2),0,cornerC(1),cornerC(2),0,wgs84Ellipsoid);
    [bNorth,bEast,bDown] = geodetic2ned(cornerB(1),cornerB(2),0,cornerC(1),cornerC(2),0,wgs84Ellipsoid);
    [cNorth,cEast,cDown] = geodetic2ned(cornerC(1),cornerC(2),0,cornerC(1),cornerC(2),0,wgs84Ellipsoid);
    [dNorth,dEast,dDown] = geodetic2ned(cornerD(1),cornerD(2),0,cornerC(1),cornerC(2),0,wgs84Ellipsoid);
    a=[aNorth;aEast;aDown];
    b=[bNorth;bEast;bDown];
    c=[cNorth;cEast;cDown];
    d=[dNorth;dEast;dDown];
    AB = b-a;
    BC = c-b;
    CD = d-c;
    DA = a-d;
    if WALL == 1
        wall_vect = AB;
        if ctrl_clockwise == true
            wall_vect2 = BC;
        else
            wall_vect2 = DA;
        end
    elseif WALL == 2
        wall_vect = BC;
        if ctrl_clockwise == true
            wall_vect2 = CD;
        else
            wall_vect2 = AB;
        end
    elseif  WALL == 3
        wall_vect = CD;
        if ctrl_clockwise == true
            wall_vect2 = DA;
        else
            wall_vect2 = BC;
        end
    else   
        wall_vect = DA;
        if ctrl_clockwise == true
            wall_vect2 = AB;
        else
            wall_vect2 = CD;
        end
    end
end

== matlab function sim_all/Controller_mk4_v3/signal_to_NED/prof_trigger ==
  settings: updateMethod=DISCRETE  sampleTime=ctrl_Ts
  data: state input; trigg_prof output
%% Trigger per la gestione dei segnali
% 1 se siamo in superficie
% 0 se siamo in profondità
function trigg_prof = fcn(state)
tmp = 0;
switch state
    case 100            % fermo in superficie
        tmp = 1;
    case 101            % orientazione verso parete di inizio in superficie
        tmp = 1;
    case 102            % posizionamento in superficie
        tmp = 1;   
    case 103            % immersione
        tmp = 1;
    case 104            % orientazione in profondità
        tmp = 0;
    case 201            % pattugliamento
        tmp = 0;
    case 202            % frenata
        tmp = 0;
    case 203            % manovra di cambio parete
        tmp = 0;
    case 204            % competamento del pattugliamento della parete iniziale
        tmp = 0;
    case 205            % frenata a metà parete
        tmp = 0;
    case 301            % risalita
        tmp = 0;
    case 302            % orientazione in superficie
        tmp = 1;
    case 303            % rientro, ritorno al punto iniziale in superficie
        tmp = 1;
    case 304            % fine missione, tutto spento
        tmp = 1;
end
trigg_prof = tmp;
end

== matlab function sim_all/EKF/Calcolo distaza pareti/Calcolo distanza dalle pareti ==
  data: pos_es input; dpp output; dps output; parete_attuale input; nav_plane_AB parameter; nav_plane_BC parameter; nav_plane_CD parameter; nav_plane_DA parameter; nav_giro parameter
% Applicando la formula della distanza di un punto da un piano si ottiene la
% distanza della posizione dell'AUV dalla parete d'interesse. 

function [dpp,dps] = dpp_dps_calculator(pos_es, parete_attuale, nav_plane_AB, nav_plane_BC, nav_plane_CD, nav_plane_DA, nav_giro)
    
%selezione della parete di pattugliamento e successiva
    switch parete_attuale
        
        case 1
           coef = nav_plane_AB;            %parete attuale AB
           if nav_giro == 1
               coef_succ = nav_plane_BC;   %parete succ BC
           else
               coef_succ = nav_plane_DA;   %parete succ DA
           end
           
        case 2
           coef = nav_plane_BC;            %parete attuale BC
           if nav_giro == 1
               coef_succ = nav_plane_CD;   %parete succ CD
           else
               coef_succ = nav_plane_AB;   %parete succ AB
           end
           
        case 3
           coef = nav_plane_CD;            %parete attuale CD
           if nav_giro == 1
               coef_succ = nav_plane_DA;   %parete succ DA
           else
               coef_succ = nav_plane_BC;   %parete succ BC
           end
        case 4
           coef = nav_plane_DA;            %parete attuale DA
           if nav_giro == 1
               coef_succ = nav_plane_AB;   %parete succ AB
           else
               coef_succ = nav_plane_CD;   %parete succ CD
           end
        otherwise
            coef = [0 0 0 0];
            coef_succ = [0 0 0 0];
    end

    dpp = abs(coef(1)*pos_es(1)+coef(2)*pos_es(2)-coef(3)*pos_es(3)+coef(4))/norm([coef(1) coef(2) coef(3)]);
    dps = abs(coef_succ(1)*pos_es(1)+coef_succ(2)*pos_es(2)-coef_succ(3)*pos_es(3)+coef_succ(4))/norm([coef_succ(1) coef_succ(2) coef_succ(3)]);
   
end
